simulink library "cam"  (R2023b)
settings: Solver=VariableStepAuto  StartTime=0.0  StopTime=10.0  RelTol=1e-3
undefined symbols (not defined in the file): cam_focale, cam_fps, cam_l, cam_noise, cam_position, cam_q, cam_res
libraries: accelerometers x6, simulink x1
settings Model: Creator=robin  LastModifiedBy=robin

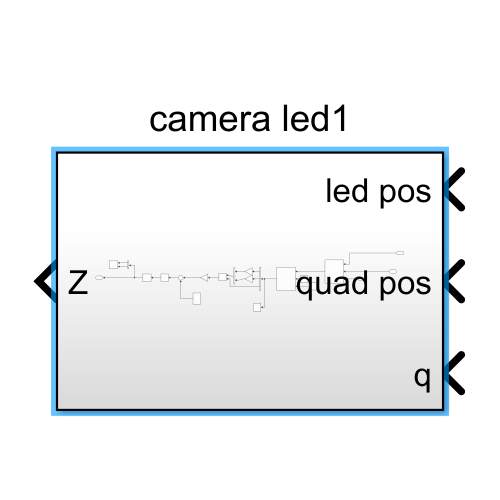
[thumbnail: Simulink's stored preview of the top-level diagram]
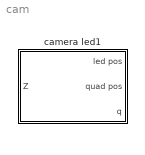
== system cam ==
  camera led1 : Subsystem

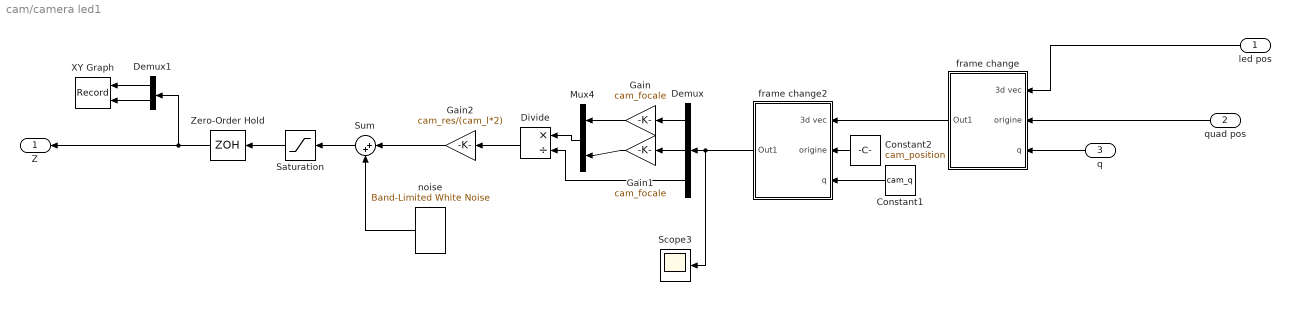
== system cam/camera led1 ==
  led pos : Inport
  quad pos : Inport  Port=2
  q : Inport  Port=3
  Constant1 : Constant  Value=cam_q
  Constant2 : Constant  Value=cam_position
  Demux : Demux  Outputs=3
  Demux1 : Demux  Outputs=2
  Divide : Product  Inputs=*/
  Gain : Gain  Gain=cam_focale
  Gain1 : Gain  Gain=cam_focale
  Gain2 : Gain  Gain=cam_res/(cam_l*2)
  Mux4 : Mux  Inputs=2
  Saturation : Saturate  UpperLimit=0.5*cam_res  LowerLimit=-0.5*cam_res  LinearizeAsGain=off
  Scope3 : Scope
  Sum : Sum  Inputs=|++
  XY Graph : Record  FileSettingsInternal="{\"entries\":[{\"content\":{\"excelSettings\":{\"content\":{},\"type\":\"Streamout.ExcelSettings\"}},\"type\":\"Streamout.FileSettingStorage\",\"uuid\":\"\"}],\"packageUris\":[\"http:\\/\\/schema.mathworks.com\\/mf0\\/streamout_blocks\\/R2020a\"],\"version\":\"1.0\"}"  Layout=[1 1]  SignalsInternal="{\"entries\":[{\"content\":{\"signals\":[{\"content\":{\"blockPath\":[],\"dimensions\":[1,1],\"domain\":\"\",\"lineColor\":\"#ff6929\",\"port\":1,\"signalID\":24,\"signalName\":\"Demux1:1\"},\"type\":\"RecordBlkView.Signal\",\"uuid\":\"\"},{\"content\":{\"blockPath\":[],\"dimensions\":[1,1],\"domain\":\"\",\"lineColor\":\"#b746ff\",\"port\":2,\"signalID\":27,\"signalName\":\"Demux1:2\"},\"type\":\"RecordBlkView.Signal\",\"uuid\":\"\"}]},\"type\":\"RecordBlkView.InputSignals\",\"uuid\":\"\"}],\"packageUris\":[\"http:\\/\\/schema.mathworks.com\\/mf0\\/streamout_blocks\\/R2020a\"],\"version\":\"1.0\"}"  VisualizationBindings="{\"xyplotplugin\":{\"info\":[{\"series\":[],\"subplotID\":1}]}}"  CompatibilityTag=XY
  Zero-Order Hold : ZeroOrderHold  SampleTime=1/cam_fps
  frame change : Subsystem
  frame change2 : Subsystem
  noise : simulink/Sources/Band-Limited White Noise  Cov="[(pi*cam_noise/cam_fps)^2  (pi*cam_noise/cam_fps)^2 ]"  Ts=1/cam_fps  seed=[randi(1020) randi(1030)]  VectorParams1D=off
  Z : Outport
  wires:
  frame change/1(Out1) -> frame change2/1(3d vec)
  q/1 -> frame change/3(q)
  Demux/3 -> Divide/2
  Demux/2 -> Gain1/1
  Constant1/1 -> frame change2/3(q)
  frame change2/1(Out1) -> Scope3/1, Demux/1
  Demux/1 -> Gain/1
  Demux1/1 -> XY Graph/1
  Divide/1 -> Gain2/1
  Mux4/1 -> Divide/1
  Gain1/1 -> Mux4/2
  Gain/1 -> Mux4/1
  Sum/1 -> Saturation/1
  noise/1 -> Sum/2
  Demux1/2 -> XY Graph/2
  Gain2/1 -> Sum/1
  Constant2/1 -> frame change2/2(origine)
  Saturation/1 -> Zero-Order Hold/1
  quad pos/1 -> frame change/2(origine)
  led pos/1 -> frame change/1(3d vec)
  Zero-Order Hold/1 -> Demux1/1, Z/1

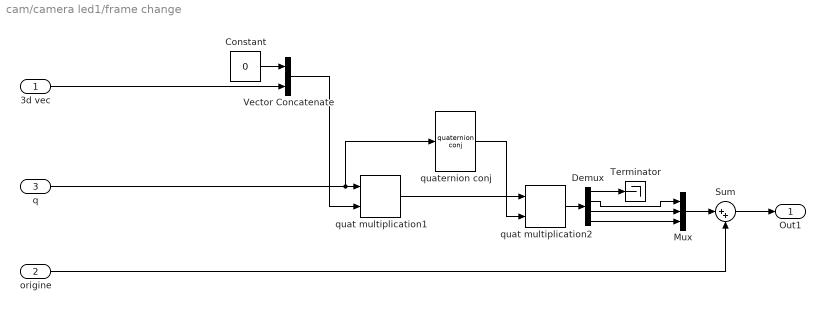
== system cam/camera led1/frame change ==
  3d vec : Inport
  origine : Inport  Port=2
  q : Inport  Port=3
  Constant : Constant  Value=0
  Demux : Demux
  Mux : Mux  Inputs=3
  Sum : Sum  Inputs=|++
  Terminator : Terminator
  Vector Concatenate : Concatenate
  quat multiplication1 : accelerometers/accelerometer/quat multiplication1  SystemSampleTime=-1  VariantActivationTime=update diagram  AllowFlexibleInterface=on  Latency=0  AutoFrameSizeCalculation=off
  quat multiplication2 : accelerometers/accelerometer/quat multiplication2  SystemSampleTime=-1  VariantActivationTime=update diagram  AllowFlexibleInterface=on  Latency=0  AutoFrameSizeCalculation=off
  quaternion conj : accelerometers/accelerometer/quaternion conj  SystemSampleTime=-1  VariantActivationTime=update diagram  AllowFlexibleInterface=on  Latency=0  AutoFrameSizeCalculation=off
  Out1 : Outport
  wires:
  Demux/1 -> Terminator/1
  Vector Concatenate/1 -> quat multiplication1/2
  quaternion conj/1 -> quat multiplication2/2
  quat multiplication2/1 -> Demux/1
  Constant/1 -> Vector Concatenate/1
  q/1 -> quaternion conj/1, quat multiplication1/1
  quat multiplication1/1 -> quat multiplication2/1
  Demux/3 -> Mux/2
  Demux/4 -> Mux/3
  Demux/2 -> Mux/1
  3d vec/1 -> Vector Concatenate/2
  Mux/1 -> Sum/1
  Sum/1 -> Out1/1
  origine/1 -> Sum/2

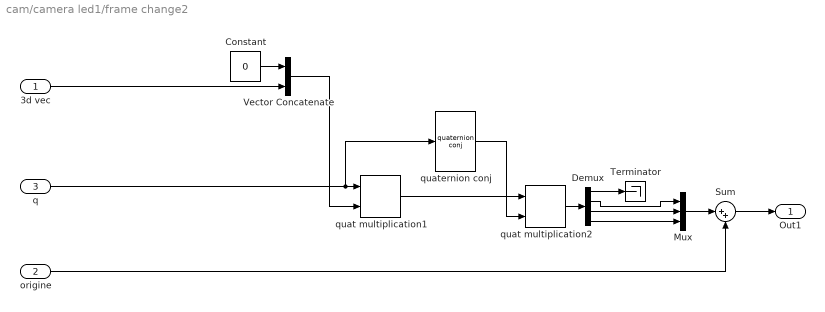
== system cam/camera led1/frame change2 ==
  3d vec : Inport
  origine : Inport  Port=2
  q : Inport  Port=3
  Constant : Constant  Value=0
  Demux : Demux
  Mux : Mux  Inputs=3
  Sum : Sum  Inputs=|++
  Terminator : Terminator
  Vector Concatenate : Concatenate
  quat multiplication1 : accelerometers/accelerometer/quat multiplication1  SystemSampleTime=-1  VariantActivationTime=update diagram  AllowFlexibleInterface=on  Latency=0  AutoFrameSizeCalculation=off
  quat multiplication2 : accelerometers/accelerometer/quat multiplication2  SystemSampleTime=-1  VariantActivationTime=update diagram  AllowFlexibleInterface=on  Latency=0  AutoFrameSizeCalculation=off
  quaternion conj : accelerometers/accelerometer/quaternion conj  SystemSampleTime=-1  VariantActivationTime=update diagram  AllowFlexibleInterface=on  Latency=0  AutoFrameSizeCalculation=off
  Out1 : Outport
  wires:
  Demux/1 -> Terminator/1
  Vector Concatenate/1 -> quat multiplication1/2
  quaternion conj/1 -> quat multiplication2/2
  quat multiplication2/1 -> Demux/1
  Constant/1 -> Vector Concatenate/1
  q/1 -> quaternion conj/1, quat multiplication1/1
  quat multiplication1/1 -> quat multiplication2/1
  Demux/3 -> Mux/2
  Demux/4 -> Mux/3
  Demux/2 -> Mux/1
  3d vec/1 -> Vector Concatenate/2
  Mux/1 -> Sum/1
  Sum/1 -> Out1/1
  origine/1 -> Sum/2
